simulink model "DenoisingProcedure"  (R2024b)
settings: Solver=FixedStepAuto  StartTime=0.0  StopTime=10  FixedStep=0.0001  RelTol=1e-3
undefined symbols (not defined in the file or in its folder): dspblkCoreblockFVToolHelper, gcbh, Ts
libraries: dspspect3 x3, dspsigops x2, dspxfrm3 x1
settings Model: Creator=Caohuaqi  LastModifiedBy=Caohuaqi

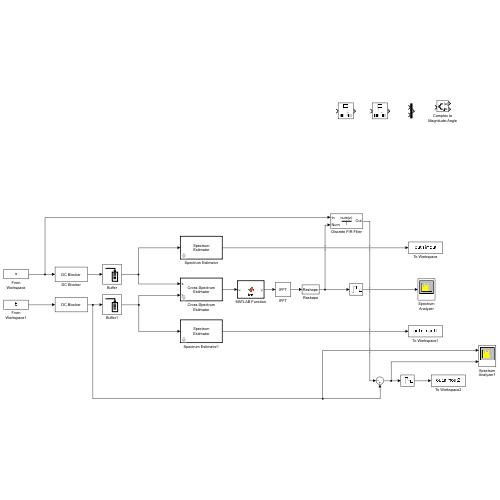
[thumbnail: Simulink's stored preview of the top-level diagram]
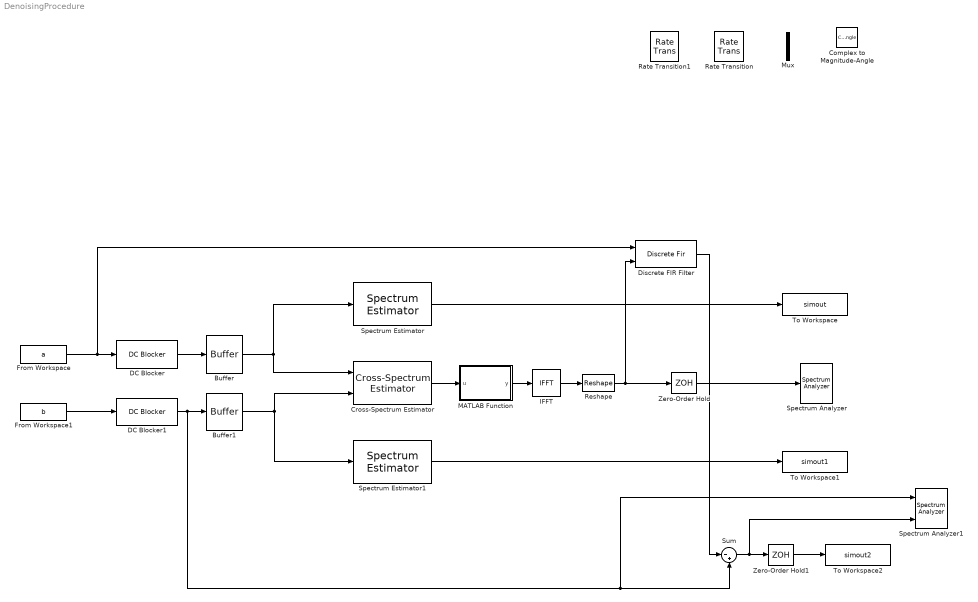
== system DenoisingProcedure ==
  Buffer : Buffer  N=10000  V=50  OutputFrames=off
  Buffer1 : Buffer  N=10000  V=50  OutputFrames=off
  Complex to Magnitude-Angle : ComplexToMagnitudeAngle
  Cross-Spectrum Estimator : dspspect3/Cross-Spectrum Estimator  WindowLength=1024  Overlap=50  AveragingMethod=Running  ForgettingFactorPort=off  ForgettingFactor=0.9  SpectralAverages=1  FFTLengthSource=Auto  FFTLength=128  Window=Hamming  SidelobeAttenuation=60  FrequencyRange=Centered  InheritSampleRate=on  SampleRate=44100  SimulateUsing=Interpreted execution
  DC Blocker : dspsigops/DC Blocker  Algorithm=IIR  NormalizedBandwidth=0.001  Length=50  Order=6  SimulateUsing=Interpreted execution
  DC Blocker1 : dspsigops/DC Blocker  Algorithm=IIR  NormalizedBandwidth=0.001  Length=50  Order=6  SimulateUsing=Interpreted execution
  Discrete FIR Filter : DiscreteFir  LoadFcn=dspblkCoreblockFVToolHelper(gcbh,'load');  CoefSource=Input port
      settings: CopyFcn=dspblkCoreblockFVToolHelper(gcbh,'copy');  DeleteFcn=dspblkCoreblockFVToolHelper(gcbh,'close');  ModelCloseFcn=dspblkCoreblockFVToolHelper(gcbh,'close');  PreSaveFcn=dspblkCoreblockFVToolHelper(gcbh,'presave');  PostSaveFcn=dspblkCoreblockFVToolHelper(gcbh,'postsave');  CloseFcn=dspblkCoreblockFVToolHelper(gcbh,'close');  InputPortMap=u0,u1
  From Workspace : FromWorkspace  VariableName=a  SampleTime=Ts  ZeroCross=off  OutputAfterFinalValue=Holding final value
  From Workspace1 : FromWorkspace  VariableName=b  SampleTime=Ts  OutputAfterFinalValue=Holding final value
  IFFT : dspxfrm3/IFFT  FFTImplementation=Auto  CompMethod=Table lookup  TableOpt=NEW  TableOptActive=Speed  BitRevOrder=off  cs_in=off  Normalize=on  InheritFFTLength=on  FFTLength=64  WrapInput=on  mode=Real  outSamplingMode=Sample based  roundingMode=Ceiling  overflowMode=off  firstCoeffDataTypeStr=Inherit: Same word length as input  firstCoeffLastDataTypeStr=Inherit: Same word length as input  outputMin=[]  outputMax=[]
  MATLAB Function : MATLAB Function  TreatAsAtomicUnit=on
  Mux : Mux  Inputs=2
  Rate Transition : RateTransition  OutPortSampleTime=0.0002
  Rate Transition1 : RateTransition  OutPortSampleTime=0.0002
  Reshape : Reshape  OutputDimensionality=Customize  OutputDimensions=[10000,1]
  Spectrum Analyzer : SpectrumAnalyzer  WindowPosition=[330.000000,251.000000,1028.000000,757.000000,]  ScopeFrameLocation=window  SampleRateSource=Property  SampleRate=5000  WindowInvariantSamplesPerUpdate=on  Span=5000  StartFrequency=-2500  StopFrequency=2500  YLimits=[-207.49579297,-120.8698934]
  Spectrum Analyzer1 : SpectrumAnalyzer  NumInputPorts=2  WindowPosition=[330.000000,251.000000,1028.000000,757.000000,]  Visible=on  ScopeFrameLocation=window  InputDomain=Frequency  SampleRateSource=Property  SampleRate=5000  WindowInvariantSamplesPerUpdate=on  Span=5000  StartFrequency=-2500  StopFrequency=2500  SpectrumUnits=Auto  YLimits=[-72.80017622,16.4414349]  SelectedToolstripTab=spectrumAnalyzerToolstrip.estimationTab
  Spectrum Estimator : dspspect3/Spectrum Estimator  Method=Filter bank  NumTapsPerBand=12  SpectrumType=Power  FrequencyResolutionMethod=Auto  FilterBankResolutionMethod=Auto  RBW=5  WindowLength=1024  FrequencyBandsSource=Same as input frame size  FrequencyBands=1024  FFTLengthSource=Auto  FFTLength=1024  InheritSampleRate=on  SampleRate=44100  Window=Hann  SidelobeAttenuation=60  AveragingMethod=Exponential  SpectralAverages=1  ForgettingFactorPort=off  ForgettingFactor=0.9  Overlap=0  ReferenceLoad=1  FrequencyRange=Centered  PowerUnits=dBm  SimulateUsing=Interpreted execution  OutputMaxHoldSpectrum=off  OutputMinHoldSpectrum=off  OutputFrequencyVector=off  OutputRBW=off
  Spectrum Estimator1 : dspspect3/Spectrum Estimator  Method=Filter bank  NumTapsPerBand=12  SpectrumType=Power  FrequencyResolutionMethod=Auto  FilterBankResolutionMethod=Auto  RBW=5  WindowLength=1024  FrequencyBandsSource=Same as input frame size  FrequencyBands=1024  FFTLengthSource=Auto  FFTLength=1024  InheritSampleRate=on  SampleRate=44100  Window=Hann  SidelobeAttenuation=60  AveragingMethod=Exponential  SpectralAverages=1  ForgettingFactorPort=off  ForgettingFactor=0.9  Overlap=0  ReferenceLoad=1  FrequencyRange=Centered  PowerUnits=dBm  SimulateUsing=Interpreted execution  OutputMaxHoldSpectrum=off  OutputMinHoldSpectrum=off  OutputFrequencyVector=off  OutputRBW=off
  Sum : Sum  Inputs=|-+
  To Workspace : ToWorkspace  VariableName=simout  SaveFormat=Timeseries  SampleTime=-1
  To Workspace1 : ToWorkspace  VariableName=simout1  SaveFormat=Timeseries  SampleTime=-1
  To Workspace2 : ToWorkspace  VariableName=simout2  SaveFormat=Timeseries  SampleTime=-1
  Zero-Order Hold : ZeroOrderHold  SampleTime=Ts
  Zero-Order Hold1 : ZeroOrderHold  SampleTime=Ts
  wires:
  Buffer/1 -> Spectrum Estimator/1, Cross-Spectrum Estimator/1
  Buffer1/1 -> Cross-Spectrum Estimator/2, Spectrum Estimator1/1
  Spectrum Estimator/1 -> To Workspace/1
  Spectrum Estimator1/1 -> To Workspace1/1
  DC Blocker/1 -> Buffer/1
  DC Blocker1/1 -> Spectrum Analyzer1/1, Sum/2, Buffer1/1
  MATLAB Function/1(y) -> IFFT/1
  Discrete FIR Filter/1 -> Sum/1
  Cross-Spectrum Estimator/1 -> MATLAB Function/1(u)
  IFFT/1 -> Reshape/1
  Reshape/1 -> Zero-Order Hold/1, Discrete FIR Filter/2
  Sum/1 -> Spectrum Analyzer1/2, Zero-Order Hold1/1
  Zero-Order Hold1/1 -> To Workspace2/1
  Zero-Order Hold/1 -> Spectrum Analyzer/1
  From Workspace/1 -> Discrete FIR Filter/1, DC Blocker/1
  From Workspace1/1 -> DC Blocker1/1

== matlab function DenoisingProcedure/MATLAB Function ==
  data: u input; y output
function y = fcn(u)

y = u;
